simulink model "feed_system_harness_fuel_hotfire"  (R2025b)
settings: Solver=ode23t  StartTime=0  StopTime=8  RelTol=1e-3
undefined symbols (not defined in the file or in its folder): eregValveDelay, fuelClose, fuelCracking, fuelMdot, fuelOpen, fuelRho, fuelSetpoint, KcFuel, Kp1Fuel, Kp2Fuel, KpRampTimeFuel, linearFitFuel, mainValveTime, modelName, OFRatio, T_prop_n2
libraries: fl_lib x11, nesl_utility x7, simulink x4
(part 2 of 2)

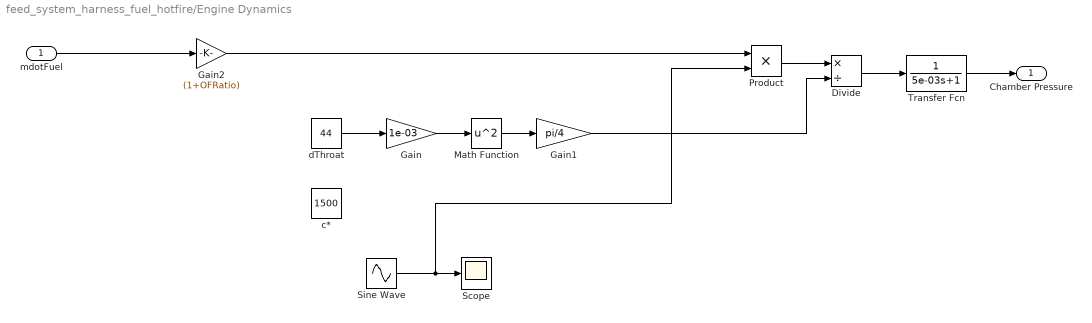
== system feed_system_harness_fuel_hotfire/Engine Dynamics ==
  mdotFuel : Inport
  Divide : Product  Inputs=*/
  Gain : Gain  Gain=1e-03
  Gain1 : Gain  Gain=pi/4
  Gain2 : Gain  Gain=(1+OFRatio)
  Math Function : Math  Operator=square
  Product : Product
  Scope : Scope
      settings: ActiveDisplayYMinimum=1312.500487492101  ActiveDisplayYMaximum=1687.4998929895169
  Sine Wave : Sin  Amplitude=100  Bias=1400  Frequency=10  Phase=pi  SampleTime=0.005
  Transfer Fcn : TransferFcn  Denominator=[5e-03 1]
  c* : Constant  Value=1500
  dThroat : Constant  Value=44
  Chamber Pressure : Outport
  wires:
  dThroat/1 -> Gain/1
  Gain/1 -> Math Function/1
  Math Function/1 -> Gain1/1
  Product/1 -> Divide/1
  Gain1/1 -> Divide/2
  Divide/1 -> Transfer Fcn/1
  Transfer Fcn/1 -> Chamber Pressure/1
  mdotFuel/1 -> Gain2/1
  Gain2/1 -> Product/1
  Sine Wave/1 -> Product/2, Scope/1

== matlab function feed_system_harness_fuel_hotfire/FeedBack Command ==
  data: propPressure input; propSetpoint input; valveAngle output; nd_error output; Kp input; fuelOpen input; fuelCracking input
function [valveAngle, nd_error] = eregControl(propPressure, propSetpoint, Kp, fuelOpen, fuelCracking)
nd_error = (1 - propPressure/propSetpoint); %Non dimensional error

valveAngle = nd_error * (fuelOpen - fuelCracking) * Kp;

== matlab function feed_system_harness_fuel_hotfire/FeedForwardCommand Fuel ==
  data: n2Pressure input; valveAngle output; CdA_measured output; CdACorrectionFactor input; linearFitFuel input; mdotProp input; rhoProp input; CdA output
function [valveAngle, CdA_measured, CdA] = feedForwardAngle(n2Pressure, CdACorrectionFactor, linearFitFuel, mdotProp, rhoProp)
    % Required effective flow area
    CdA_measured = (mdotProp / rhoProp) * 1/sqrt(max(0,n2Pressure)) * 0.673;
    CdA = CdA_measured * CdACorrectionFactor;
    
    valveAngle = max(polyval(linearFitFuel,CdA));

end

== matlab function feed_system_harness_fuel_hotfire/CdA Robustness Function ==
  data: array output; shiftBool input; shiftIdx input; scaleFactor input
function array = CdAArray(shiftBool, shiftIdx, scaleFactor)
array   = [0, 0, 0, 4.0e-6, 12.7e-6, 15.2e-6, 17.1e-6, 18.6e-6, 19.5e-6, 19.8e-6];
array = array * scaleFactor;
if shiftBool == true
    array = shiftArray(array, shiftIdx);
end

end

function shifted = shiftArray(array, n)
    % Shifts array by n positions.
    %   n > 0: shifts forward (right), padding the start with the first value
    %   n < 0: shifts backward (left), padding the end with the last value
    %   n = 0: returns array unchanged

    N = numel(array);
    shifted = zeros(size(array));

    if n >= 0
        n = min(n, N);
        shifted(1:n) = array(1);                  % pad start with first value
        shifted(n+1:end) = array(1:N-n);
    else
        n = min(-n, N);
        shifted(1:N-n) = array(n+1:end);
        shifted(N-n+1:end) = array(end);           % pad end with last value
    end
end

== matlab function feed_system_harness_fuel_hotfire/MATLAB Function ==
  data: u input; y output; fuelClose input; fuelOpen input
function y = fcn(u, fuelClose, fuelOpen)

y = (u - fuelClose)/(fuelOpen - fuelClose);
